simulink model "Velo_BO_Moteur"  (R2018a)
settings: Solver=VariableStepAuto  StartTime=0.0  StopTime=simTime  RelTol=1e-3
undefined symbols (not defined in the file): AccelVal, AngleInitial
libraries: simulink x1
settings Model: Creator=chsira  LastModifiedBy=charl
settings DebuggingCC: LibraryContextMissingDiagnostic=warning
settings SFSimCC: SimUseLocalCustomCode=on
settings RTWCC: RTWUseLocalCustomCode=on

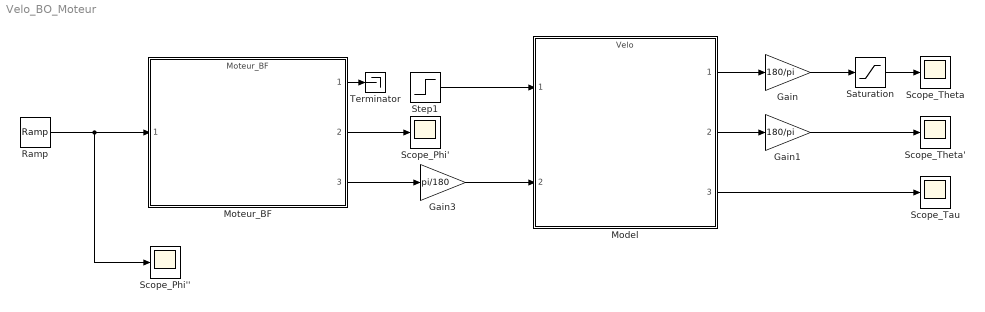
== system Velo_BO_Moteur ==
  Gain : Gain  Gain=180/pi
  Gain1 : Gain  Gain=180/pi
  Gain3 : Gain  Gain=pi/180
  Model : ModelReference  ModelNameDialog=Velo.slx  ParameterArgumentNames=InitialCondition  ParameterArgumentValues=InitialCondition  UsingDefaultArgumentValue=0  SimulationMode=Normal  ModelReferenceVersion=1.73  InitialCondition=AngleInitial*pi/180  SimulationMode=Normal
  "Moteur_BF " : ModelReference  ModelNameDialog=Moteur_BF  SimulationMode=Normal  ModelReferenceVersion=1.78
  Ramp : simulink/Sources/Ramp  slope=AccelVal  start=0  InitialOutput=0
  Saturation : Saturate  UpperLimit=20  LowerLimit=-20
  "Scope_Phi' " : Scope
  Scope_Phi'' : Scope
  Scope_Tau : Scope
  Scope_Theta : Scope
  Scope_Theta' : Scope
  Step1 : Step  Time=0  After=0  SampleTime=0
  Terminator : Terminator
  wires:
  Model/3 -> Scope_Tau/1
  Model/2 -> Gain1/1
  Model/1 -> Gain/1
  Gain1/1 -> Scope_Theta'/1
  Gain/1 -> Saturation/1
  Saturation/1 -> Scope_Theta/1
  Step1/1 -> Model/1
  Gain3/1 -> Model/2
  "Moteur_BF "/3 -> Gain3/1
  Ramp/1 -> Scope_Phi''/1, "Moteur_BF "/1
  "Moteur_BF "/2 -> "Scope_Phi' "/1
  "Moteur_BF "/1 -> Terminator/1
